simulink model "sim_quadrotor"  (R2015a)
settings: Solver=ode3  StartTime=0  StopTime=40  FixedStep=sampleTime_qcsim  MaxStep=0.1  RelTol=1e-3
InitFcn:
  | % load parameters of the default quadrotor
  | disp('Quadrotor parameters loaded by InitFcn')
  | paramsFilters %load mdl_quadcopter as well!
  | 
  | % change to Simulation folder if in data folder
  | cd([matlabpath '/Simulation']);
values from neighbouring files (symbols this model uses):
  K_lqr_toMotorcmd = lqr(A,B,Q,R)    [LQRControl.m]
undefined symbols (not defined in the file or in its folder): altEstim, controlParams, Discrete, K_poleplace, ofhandle, quad, quadEDT, sampleTime_qcsim, Time, vishandle
libraries: simulink x29, ctrlSharedLib x3, commnoisgen2 x1
(part 2 of 2)

== system sim_quadrotor/DroneRS_Compensator/ControllerFSFB/SysteminputConverter/Takeoffphase_Thrustadjustment ==
  note: NOTE: Below 40cm in altitude, sonar measurements and camera data are very unreliable.
      | We therefore introduce a take-off phase where the drone controls attitude only and runs an uncontrolled total thrust of takeofff_Gain/100  % above equilibrium thrust.
  takeoffphase_flagin : Inport
  totThrustbyController_refin : Inport  Port=2
  Add1 : Sum  Inputs=++|
  HoverThrustLinearizationPoint : Constant  Value=-quad.g*quad.M
  "SCOPE_totalthrust " : Scope
  SaturationThrust : Saturate  UpperLimit=controlParams.totalThrust_maxRelative*controlParams.motorsThrust_i_UpperLimit*4  LowerLimit=-(controlParams.totalThrust_maxRelative*controlParams.motorsThrust_i_UpperLimit*4)
  TakeoffOrControl_Switch : Switch  Criteria=u2 > Threshold
  takeoff_Gain : Gain  Gain=controlParams.takeoff_Gain
  totThrust_refout : Outport
  wires:
  takeoffphase_flagin/1 -> TakeoffOrControl_Switch/2
  SaturationThrust/1 -> totThrust_refout/1, "SCOPE_totalthrust "/1
  TakeoffOrControl_Switch/1 -> Add1/2
  takeoff_Gain/1 -> TakeoffOrControl_Switch/1
  HoverThrustLinearizationPoint/1 -> Add1/1, takeoff_Gain/1
  totThrustbyController_refin/1 -> TakeoffOrControl_Switch/3
  Add1/1 -> SaturationThrust/1

== system sim_quadrotor/DroneRS_Compensator/ControllerFSFB/SysteminputConverter/Thrust2Motorcmd ==
  note: NOTE: This block translates thrust per motor into a command that is acutally send to the motors.
  thrust_refin : Inport
  MotorsRotationDirection : Gain  Gain=[-1,1,-1,1]
  Signed Sqrt : Sqrt  Operator=signedSqrt  SaturateOnIntegerOverflow=on
  ThrustToW2_Gain : Gain  Gain=1/(quad.Ct*quad.rho*quad.A*quad.r^2)
  W2ToMotorsCmd_Gain : Gain  Gain=1/quadEDT.motorsRSToW2_Gain
  motors_cmdout : Outport
  wires:
  MotorsRotationDirection/1 -> W2ToMotorsCmd_Gain/1, Signed Sqrt/1
  Signed Sqrt/1 -> ?  "w"
  W2ToMotorsCmd_Gain/1 -> motors_cmdout/1
  thrust_refin/1 -> ThrustToW2_Gain/1
  ThrustToW2_Gain/1 -> MotorsRotationDirection/1

== system sim_quadrotor/DroneRS_Compensator/ControllerLQR/SysteminputConverter/ControlMixerRS ==
  note: NOTE: The controlmixer translates total thrust and the three torque inputs that the controller came up with into 'thrust per motor'.
  T_refin : Inport
  Qyaw_refin : Inport  Port=2
  Qpitch_refin : Inport  Port=3
  Qroll_refin : Inport  Port=4
  Mux2 : Mux
  Product : Product  Multiplication=Matrix(*)  RndMeth=Zero
  Saturation2 : Saturate  UpperLimit=-0.0118  LowerLimit=-0.3235
  TorquetotalThrustToThrustperMotor : Constant  Value=controlParams.Q2Ts
  thrust_refout : Outport
  wires:
  Qroll_refin/1 -> Mux2/4
  Qpitch_refin/1 -> Mux2/3
  Qyaw_refin/1 -> Mux2/2
  T_refin/1 -> Mux2/1
  Product/1 -> Saturation2/1
  TorquetotalThrustToThrustperMotor/1 -> Product/1
  Mux2/1 -> Product/2
  Saturation2/1 -> thrust_refout/1

== system sim_quadrotor/DroneRS_Compensator/ControllerLQR/SysteminputConverter/Conversion Motorcommands To TotalThrust and Torques ==
  motors_cmdin : Inport
  MotorsRotationDirection : Gain  Gain=diag([-1,1,-1,1])  Multiplication=Matrix(K*u)
  ThrustperMotor To TotalThrust and Torques : Gain  Gain=controlParams.Ts2Q  Multiplication=Matrix(K*u)
  W2ToThrust : Gain  Gain=quad.Ct*quad.rho*quad.A*quad.r^2
  motorsRSToW2_Gain : Gain  Gain=quadEDT.motorsRSToW2_Gain
  u_tthrust_torques : Outport
  wires:
  ThrustperMotor To TotalThrust and Torques/1 -> u_tthrust_torques/1
  motors_cmdin/1 -> MotorsRotationDirection/1
  W2ToThrust/1 -> ThrustperMotor To TotalThrust and Torques/1
  motorsRSToW2_Gain/1 -> W2ToThrust/1
  MotorsRotationDirection/1 -> motorsRSToW2_Gain/1

== system sim_quadrotor/DroneRS_Compensator/ControllerLQR/SysteminputConverter/Takeoffphase_Thrustadjustment ==
  note: NOTE: Below 40cm in altitude, sonar measurements and camera data are very unreliable.
      | We therefore introduce a take-off phase where the drone controls attitude only and runs an uncontrolled total thrust of takeofff_Gain/100  % above equilibrium thrust.
  takeoffphase_flagin : Inport
  totThrustbyController_refin : Inport  Port=2
  Add1 : Sum  Inputs=++|
  HoverThrustLinearizationPoint : Constant  Value=-quad.g*quad.M
  "SCOPE_totalthrust " : Scope
  SaturationThrust : Saturate  UpperLimit=controlParams.totalThrust_maxRelative*controlParams.motorsThrust_i_UpperLimit*4  LowerLimit=-(controlParams.totalThrust_maxRelative*controlParams.motorsThrust_i_UpperLimit*4)
  TakeoffOrControl_Switch : Switch  Criteria=u2 > Threshold
  takeoff_Gain : Gain  Gain=controlParams.takeoff_Gain
  totThrust_refout : Outport
  wires:
  takeoffphase_flagin/1 -> TakeoffOrControl_Switch/2
  SaturationThrust/1 -> totThrust_refout/1, "SCOPE_totalthrust "/1
  TakeoffOrControl_Switch/1 -> Add1/2
  takeoff_Gain/1 -> TakeoffOrControl_Switch/1
  HoverThrustLinearizationPoint/1 -> Add1/1, takeoff_Gain/1
  totThrustbyController_refin/1 -> TakeoffOrControl_Switch/3
  Add1/1 -> SaturationThrust/1

== system sim_quadrotor/DroneRS_Compensator/ControllerLQR/SysteminputConverter/Thrust2Motorcmd ==
  note: NOTE: This block translates thrust per motor into a command that is acutally send to the motors.
  thrust_refin : Inport
  MotorsRotationDirection : Gain  Gain=[-1,1,-1,1]
  Signed Sqrt : Sqrt  Operator=signedSqrt  SaturateOnIntegerOverflow=on
  ThrustToW2_Gain : Gain  Gain=1/(quad.Ct*quad.rho*quad.A*quad.r^2)
  W2ToMotorsCmd_Gain : Gain  Gain=1/quadEDT.motorsRSToW2_Gain
  motors_cmdout : Outport
  wires:
  MotorsRotationDirection/1 -> W2ToMotorsCmd_Gain/1, Signed Sqrt/1
  Signed Sqrt/1 -> ?  "w"
  W2ToMotorsCmd_Gain/1 -> motors_cmdout/1
  thrust_refin/1 -> ThrustToW2_Gain/1
  ThrustToW2_Gain/1 -> MotorsRotationDirection/1

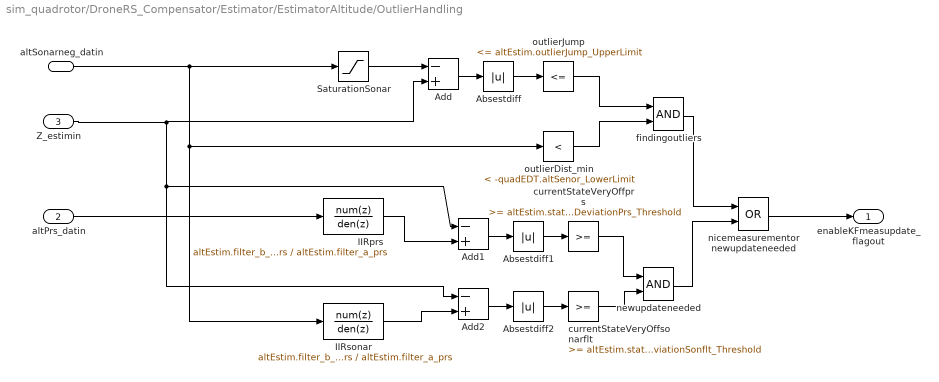
== system sim_quadrotor/DroneRS_Compensator/Estimator/EstimatorAltitude/OutlierHandling ==
  altSonarneg_datin : Inport
  altPrs_datin : Inport  Port=2
  Z_estimin : Inport  Port=3
  Absestdiff : Abs
  Absestdiff1 : Abs
  Absestdiff2 : Abs
  Add : Sum  Inputs=-+
  Add1 : Sum  Inputs=-+
  Add2 : Sum  Inputs=-+
  IIRprs : DiscreteFilter  Numerator=altEstim.filter_b_prs  Denominator=altEstim.filter_a_prs
  IIRsonar : DiscreteFilter  Numerator=altEstim.filter_b_prs  Denominator=altEstim.filter_a_prs
  SaturationSonar : Saturate  UpperLimit=-quadEDT.altSenor_LowerLimit  LowerLimit=-inf
  currentStateVeryOffprs : simulink/Logic and Bit Operations/Compare To Constant  relop=>=  const=altEstim.stateDeviationPrs_Threshold  OutDataTypeStr=boolean
  currentStateVeryOffsonarflt : simulink/Logic and Bit Operations/Compare To Constant  relop=>=  const=altEstim.stateDeviationSonflt_Threshold  OutDataTypeStr=boolean
  findingoutliers : Logic  AllPortsSameDT=off  OutDataTypeStr=boolean
  newupdateneeded : Logic  AllPortsSameDT=off  OutDataTypeStr=boolean
  nicemeasurementor newupdateneeded : Logic  Operator=OR  AllPortsSameDT=off  OutDataTypeStr=boolean
  outlierDist_min : simulink/Logic and Bit Operations/Compare To Constant  relop=<  const=-quadEDT.altSenor_LowerLimit  OutDataTypeStr=boolean
  outlierJump : simulink/Logic and Bit Operations/Compare To Constant  relop=<=  const=altEstim.outlierJump_UpperLimit  OutDataTypeStr=boolean
  enableKFmeasupdate_flagout : Outport
  wires:
  Absestdiff1/1 -> currentStateVeryOffprs/1
  IIRsonar/1 -> Add2/2
  altPrs_datin/1 -> IIRprs/1
  IIRprs/1 -> Add1/2
  currentStateVeryOffsonarflt/1 -> newupdateneeded/2
  Add2/1 -> Absestdiff2/1
  Z_estimin/1 -> Add2/1, Add1/1, Add/2
  currentStateVeryOffprs/1 -> newupdateneeded/1
  altSonarneg_datin/1 -> outlierDist_min/1, IIRsonar/1, SaturationSonar/1
  Absestdiff2/1 -> currentStateVeryOffsonarflt/1
  newupdateneeded/1 -> nicemeasurementor newupdateneeded/2
  Add/1 -> Absestdiff/1
  Absestdiff/1 -> outlierJump/1
  SaturationSonar/1 -> Add/1
  outlierJump/1 -> findingoutliers/1
  outlierDist_min/1 -> findingoutliers/2
  findingoutliers/1 -> nicemeasurementor newupdateneeded/1
  nicemeasurementor newupdateneeded/1 -> enableKFmeasupdate_flagout/1
  Add1/1 -> Absestdiff1/1

== system sim_quadrotor/DroneRS_Compensator/Estimator/EstimatorXYPosition/EstimatorVelocity ==
  opticalFlow_datin : Inport
  Z_estimin : Inport  Port=2
  sensorIMU_datin : Inport  Port=3
  att_estimin : Inport  Port=4
  AccelerationWorld : Subsystem
  Delay : Delay  DelayLength=1  InitialCondition=0
  KalmanFilter_dxdy : ctrlSharedLib/Kalman Filter  TimeDomain=Discrete-Time  UseCurrentEstimator=on  ModelSource=Individual A, B, C, D matrices  ModelSourceVariable=ss(0.95,1,1,0,1)  A=eye(2)  B=sampleTime_qcsim*eye(2)  C=eye(2)  D=0  NumberOfStates=1  NumberOfInputs=1  NumberOfOutputs=1  InitialEstimateSource=Dialog  X0=0  P0=10  UseK=off  UseGH=on  NumberOfProcessNoiseInputs=1  G=eye(2)  TimeInvariantG=on  H=0  TimeInvariantH=on  Q=0.09.*eye(2)  TimeInvariantQ=on  R=5*eye(2)  TimeInvariantR=on  N=0  TimeInvariantN=on  AddInputPort=on  AddEnablePort=on  OutputEstimatedY=off  OutputP=off  Ts=-1
  Mux : Mux  Inputs=2
  OutlierHandling : Subsystem
  SCOPEdxy : Scope
      settings: TimeRange=2.5  YMin=-12  YMax=6
  SCOPEenableKFdxupdate : Scope
      settings: TimeRange=2.2  YMin=0  YMax=1
  SelectplanarOF : Selector  InputPortWidth=3  Indices=[1 2]
  opticalFlowToVelocity_Gain : Gain  Gain=1/quadEDT.VelocityToOpticalFlow_Gain
  dxy_estimout : Outport
  wires:
  att_estimin/1 -> OutlierHandling/1(att_estimin), AccelerationWorld/1(att_estimin)
  sensorIMU_datin/1 -> AccelerationWorld/2(sensorIMU_datin), OutlierHandling/2(sensorIMU_datin)
  opticalFlow_datin/1 -> opticalFlowToVelocity_Gain/1
  SelectplanarOF/1 -> OutlierHandling/4(dxy_estimin), KalmanFilter_dxdy/2, Mux/1
  opticalFlowToVelocity_Gain/1 -> SelectplanarOF/1
  KalmanFilter_dxdy/1 -> Mux/2, dxy_estimout/1, Delay/1
  OutlierHandling/1(Enable_flag) -> SCOPEenableKFdxupdate/1, KalmanFilter_dxdy/3
  Z_estimin/1 -> OutlierHandling/3(Z_estimin)
  Mux/1 -> SCOPEdxy/1
  AccelerationWorld/1(accelerationWorld) -> KalmanFilter_dxdy/1
  Delay/1 -> OutlierHandling/5(dxyOF_datin)

== system sim_quadrotor/DroneRS_Compensator/Estimator/EstimatorXYPosition/EstimatorXYPosition ==
  dxy_estimin : Inport
  att_estimin : Inport  Port=2
  controlModePosVSAtt_flagin : Inport  Port=3
  dz_estimin : Inport  Port=4
  posVIS_datin : Inport  Port=5
  usePosVIS_flagin : Inport  Port=6
  Delay : Delay  DelayLength=1  InitialCondition=0
  KalmanFilter_posxy : ctrlSharedLib/Kalman Filter  TimeDomain=Discrete-Time  UseCurrentEstimator=on  ModelSource=Individual A, B, C, D matrices  ModelSourceVariable=ss(0.95,1,1,0,1)  A=eye(2)  B=sampleTime_qcsim*eye(2)  C=eye(2)  D=0  NumberOfStates=1  NumberOfInputs=1  NumberOfOutputs=1  InitialEstimateSource=Dialog  X0=[.1 0.0]  P0=10  UseK=off  UseGH=on  NumberOfProcessNoiseInputs=1  G=0.1*eye(2)  TimeInvariantG=on  H=0  TimeInvariantH=on  Q=0.001*eye(2)  TimeInvariantQ=on  R=0.3*eye(2)  TimeInvariantR=on  N=0  TimeInvariantN=on  AddInputPort=on  AddEnablePort=on  OutputEstimatedY=off  OutputP=off  Ts=-1
  Mux2 : Mux  Inputs=2
  OutlierHandling : Subsystem
  RStoWorld : MATLAB Function  TreatAsAtomicUnit=on
  SelectXY : Selector  InputPortWidth=4  Indices=[1 2]
  SelectdXY : Selector  InputPortWidth=3  Indices=[1 2]
  SimplyIntegrateVelocity : DiscreteIntegrator  ExternalReset=rising  InitialConditionSetting=State (most efficient)  SampleTime=sampleTime_qcsim  LimitOutput=on  UpperSaturationLimit=2  LowerSaturationLimit=-2
  UseIPPosSwitch : Switch  Criteria=u2 > Threshold
  XY_estimout : Outport
  wires:
  att_estimin/1 -> RStoWorld/1(attitude), OutlierHandling/1(att_estimin)
  dxy_estimin/1 -> Mux2/1
  SimplyIntegrateVelocity/1 -> UseIPPosSwitch/3
  dz_estimin/1 -> Mux2/2
  Mux2/1 -> RStoWorld/2(vector)
  RStoWorld/1(vel_world) -> SelectdXY/1
  SelectdXY/1 -> KalmanFilter_posxy/1, SimplyIntegrateVelocity/1
  posVIS_datin/1 -> SelectXY/1, OutlierHandling/2(posVIS_datin)
  KalmanFilter_posxy/1 -> Delay/1, UseIPPosSwitch/1
  controlModePosVSAtt_flagin/1 -> SimplyIntegrateVelocity/2
  UseIPPosSwitch/1 -> XY_estimout/1
  usePosVIS_flagin/1 -> UseIPPosSwitch/2
  SelectXY/1 -> KalmanFilter_posxy/2
  OutlierHandling/1(enable_flag) -> KalmanFilter_posxy/3
  Delay/1 -> OutlierHandling/3(pos_estim)

== system sim_quadrotor/DroneRS_Compensator/Estimator/EstimatorXYPosition/EstimatorVelocity/AccelerationWorld ==
  note: selectaccelero
  att_estimin : Inport
  sensorIMU_datin : Inport  Port=2
  Add : Sum  Inputs=-+
  Bus Selector1 : BusSelector  OutputSignals=ddx,ddy,ddz
  Mux6 : Mux  Inputs=3
  SelectPlanarddxy : Selector  InputPortWidth=3  Indices=[1 2]
  World2Body : MATLAB Function  TreatAsAtomicUnit=on
  gainaccinput : Gain  Gain=0.2
  gravity : Constant  Value=[0 0 -quad.g]
  accelerationWorld : Outport
  wires:
  att_estimin/1 -> World2Body/1(attitude)
  Bus Selector1/2 -> Mux6/2  "<ddy>"
  Mux6/1 -> Add/2
  sensorIMU_datin/1 -> Bus Selector1/1
  Bus Selector1/1 -> Mux6/1  "<ddx>"
  Bus Selector1/3 -> Mux6/3  "<ddz>"
  SelectPlanarddxy/1 -> gainaccinput/1
  gainaccinput/1 -> accelerationWorld/1
  gravity/1 -> World2Body/2(vector)
  World2Body/1(y) -> Add/1
  Add/1 -> SelectPlanarddxy/1

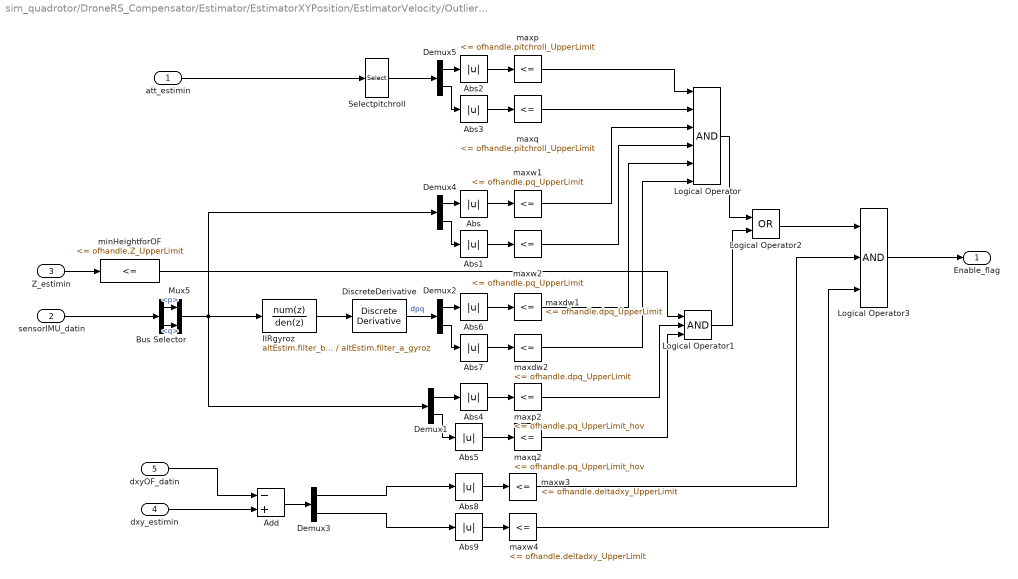
== system sim_quadrotor/DroneRS_Compensator/Estimator/EstimatorXYPosition/EstimatorVelocity/OutlierHandling ==
  att_estimin : Inport
  sensorIMU_datin : Inport  Port=2
  Z_estimin : Inport  Port=3
  dxy_estimin : Inport  Port=4
  dxyOF_datin : Inport  Port=5
  Abs{,1..9} (10 alike) : Abs
  Add : Sum  Inputs=-+
  Bus Selector : BusSelector  OutputSignals=p,q
  Demux{1..5} (5 alike) : Demux  Outputs=2
  DiscreteDerivative : simulink/Discrete/Discrete Derivative  gainval=1.0  ICPrevScaledInput=0.0  InputProcessing=Inherited  OutMin=[]  OutMax=[]  OutDataType=fixdt(1, 16)  OutScaling=2^-10  DoSatur=off
  IIRgyroz : DiscreteFilter  Numerator=altEstim.filter_b_gyroz  Denominator=altEstim.filter_a_gyroz
  Logical Operator : Logic  Inputs=6  AllPortsSameDT=off  OutDataTypeStr=boolean
  Logical Operator1 : Logic  Inputs=3  AllPortsSameDT=off  OutDataTypeStr=boolean
  Logical Operator2 : Logic  Operator=OR  AllPortsSameDT=off  OutDataTypeStr=boolean
  Logical Operator3 : Logic  Inputs=3  AllPortsSameDT=off  OutDataTypeStr=boolean
  Mux5 : Mux  Inputs=2
  Selectpitchroll : Selector  InputPortWidth=3  Indices=[2 3]
  maxdw1 : simulink/Logic and Bit Operations/Compare To Constant  relop=<=  const=ofhandle.dpq_UpperLimit  OutDataTypeStr=boolean
  maxdw2 : simulink/Logic and Bit Operations/Compare To Constant  relop=<=  const=ofhandle.dpq_UpperLimit  OutDataTypeStr=boolean
  maxp : simulink/Logic and Bit Operations/Compare To Constant  relop=<=  const=ofhandle.pitchroll_UpperLimit  OutDataTypeStr=boolean
  maxp2 : simulink/Logic and Bit Operations/Compare To Constant  relop=<=  const=ofhandle.pq_UpperLimit_hov  OutDataTypeStr=boolean
  maxq : simulink/Logic and Bit Operations/Compare To Constant  relop=<=  const=ofhandle.pitchroll_UpperLimit  OutDataTypeStr=boolean
  maxq2 : simulink/Logic and Bit Operations/Compare To Constant  relop=<=  const=ofhandle.pq_UpperLimit_hov  OutDataTypeStr=boolean
  maxw1 : simulink/Logic and Bit Operations/Compare To Constant  relop=<=  const=ofhandle.pq_UpperLimit  OutDataTypeStr=boolean
  maxw2 : simulink/Logic and Bit Operations/Compare To Constant  relop=<=  const=ofhandle.pq_UpperLimit  OutDataTypeStr=boolean
  maxw3 : simulink/Logic and Bit Operations/Compare To Constant  relop=<=  const=ofhandle.deltadxy_UpperLimit  OutDataTypeStr=boolean
  maxw4 : simulink/Logic and Bit Operations/Compare To Constant  relop=<=  const=ofhandle.deltadxy_UpperLimit  OutDataTypeStr=boolean
  minHeightforOF : simulink/Logic and Bit Operations/Compare To Constant  relop=<=  const=ofhandle.Z_UpperLimit  OutDataTypeStr=boolean
  Enable_flag : Outport
  wires:
  maxp2/1 -> Logical Operator1/2
  Demux5/2 -> Abs3/1
  minHeightforOF/1 -> Logical Operator1/1
  Demux5/1 -> Abs2/1
  maxq/1 -> Logical Operator/2
  maxdw2/1 -> Logical Operator/6
  maxdw1/1 -> Logical Operator/5
  att_estimin/1 -> Selectpitchroll/1
  maxw2/1 -> Logical Operator/4
  maxp/1 -> Logical Operator/1
  Bus Selector/2 -> Mux5/2  "<q>"
  maxq2/1 -> Logical Operator1/3
  sensorIMU_datin/1 -> Bus Selector/1
  Selectpitchroll/1 -> Demux5/1
  Bus Selector/1 -> Mux5/1  "<p>"
  maxw1/1 -> Logical Operator/3
  Logical Operator/1 -> Logical Operator2/1
  Z_estimin/1 -> minHeightforOF/1
  Abs/1 -> maxw1/1
  Abs1/1 -> maxw2/1
  Demux4/1 -> Abs/1
  Demux4/2 -> Abs1/1
  Abs2/1 -> maxp/1
  Abs3/1 -> maxq/1
  Abs4/1 -> maxp2/1
  Abs5/1 -> maxq2/1
  Demux1/1 -> Abs4/1
  Demux1/2 -> Abs5/1
  Logical Operator1/1 -> Logical Operator2/2
  Abs6/1 -> maxdw1/1
  Abs7/1 -> maxdw2/1
  Demux2/1 -> Abs6/1
  Demux2/2 -> Abs7/1
  DiscreteDerivative/1 -> Demux2/1  "dpq"
  Logical Operator3/1 -> Enable_flag/1
  Logical Operator2/1 -> Logical Operator3/1
  Abs8/1 -> maxw3/1
  Abs9/1 -> maxw4/1
  Add/1 -> Demux3/1
  dxy_estimin/1 -> Add/2
  Demux3/1 -> Abs8/1
  Demux3/2 -> Abs9/1
  dxyOF_datin/1 -> Add/1
  maxw3/1 -> Logical Operator3/2
  maxw4/1 -> Logical Operator3/3
  Mux5/1 -> Demux4/1, Demux1/1, IIRgyroz/1
  IIRgyroz/1 -> DiscreteDerivative/1

== system sim_quadrotor/DroneRS_Compensator/Estimator/EstimatorXYPosition/EstimatorXYPosition/OutlierHandling ==
  att_estimin : Inport
  posVIS_datin : Inport  Port=2
  pos_estim : Inport  Port=3
  Add1 : Sum  Inputs=+-
  Demux6 : Demux  Outputs=3
  Logical Operator3 : Logic  Inputs=4  AllPortsSameDT=off  OutDataTypeStr=boolean
  SelectX : Selector  InputPortWidth=4  Indices=[1]
  SelectXY : Selector  InputPortWidth=4  Indices=[1 2]
  abs : MATLAB Function  TreatAsAtomicUnit=on
  checkPosavailable : simulink/Logic and Bit Operations/Compare To Constant  relop=~=  const=-99  OutDataTypeStr=boolean
  maxp3 : simulink/Logic and Bit Operations/Compare To Constant  relop=<=  const=vishandle.att_UpperLimit  OutDataTypeStr=boolean
  maxq3 : simulink/Logic and Bit Operations/Compare To Constant  relop=<=  const=vishandle.att_UpperLimit  OutDataTypeStr=boolean
  planarjumpsVISPOS : simulink/Logic and Bit Operations/Compare To Constant  relop=<  const=vishandle.deltaXY  OutDataTypeStr=boolean
  enable_flag : Outport
  wires:
  att_estimin/1 -> Demux6/1
  posVIS_datin/1 -> SelectXY/1, SelectX/1
  SelectX/1 -> checkPosavailable/1
  checkPosavailable/1 -> Logical Operator3/1
  Logical Operator3/1 -> enable_flag/1
  Demux6/2 -> maxp3/1
  Demux6/3 -> maxq3/1
  maxp3/1 -> Logical Operator3/2
  maxq3/1 -> Logical Operator3/3
  SelectXY/1 -> Add1/1
  Add1/1 -> abs/1(vec)
  pos_estim/1 -> Add1/2
  abs/1(y) -> planarjumpsVISPOS/1
  planarjumpsVISPOS/1 -> Logical Operator3/4

== matlab function sim_quadrotor/Drone_Sensorsystem/camera/trafo_RTB2RSSensors_trans ==
  data: u input; y output
function y = fcn(u)
%inverse yaw-rotation
y = ([cos(pi/4) sin(pi/4) 0 ; -sin(pi/4) cos(pi/4) 0; 0 0 1]*u);

== matlab function sim_quadrotor/DroneRS_Compensator/ControllerPID2W/inverse rotation Function ==
  data: u input; y output
function y = fcn(u)
%inverse yaw-rotation
y = ([cos(u) sin(u); -sin(u) cos(u)]);

== matlab function sim_quadrotor/Drone_Sensorsystem/IMU_Pressure/trafo_RTB2RSSensors_trans ==
  data: u input; y output
function y = fcn(u)
%inverse yaw-rotation
y = ([cos(pi/4) sin(pi/4) 0 ; -sin(pi/4) cos(pi/4) 0; 0 0 1]*u);

== matlab function sim_quadrotor/Drone_Sensorsystem/IMU_Pressure/trafo_RTB2World_trans ==
  data: attitude input; vector input; y output
function y = fcn(attitude,vector)

yaw = attitude(1);
pitch = attitude(2);
roll = attitude(3);

R_RTBBody2Global =[ [ cos(pitch)*cos(yaw), cos(yaw)*sin(pitch)*sin(roll) - cos(roll)*sin(yaw), sin(roll)*sin(yaw) + cos(roll)*cos(yaw)*sin(pitch)];
[ cos(pitch)*sin(yaw), cos(roll)*cos(yaw) + sin(pitch)*sin(roll)*sin(yaw), cos(roll)*sin(pitch)*sin(yaw) - cos(yaw)*sin(roll)];
[         -sin(pitch),                               cos(pitch)*sin(roll),                               cos(pitch)*cos(roll)]];

% Rw_Global2RTBBody  = [0        sin(roll)          cos(roll);             %inverted Wronskian
%           0        cos(roll)*cos(pitch) -sin(roll)*cos(pitch);
%           cos(pitch) sin(roll)*sin(pitch) cos(roll)*sin(pitch)] / cos(pitch);
      
      
      
 y = R_RTBBody2Global*vector;      
      
%y = -([cos(pi/4) sin(pi/4); -sin(pi/4) cos(pi/4)]*u);

== matlab function sim_quadrotor/Drone_Sensorsystem/IMU_Pressure/trafo_World2RTB_trans1 ==
  data: attitude input; vector input; y output
function y = fcn(attitude,vector)

yaw = attitude(1);
pitch = attitude(2);
roll = attitude(3);

R_Global2RTBBody = [[                                cos(pitch)*cos(yaw),                                cos(pitch)*sin(yaw),          -sin(pitch)];
                    [ cos(yaw)*sin(pitch)*sin(roll) - cos(roll)*sin(yaw), cos(roll)*cos(yaw) + sin(pitch)*sin(roll)*sin(yaw), cos(pitch)*sin(roll)];
                    [ sin(roll)*sin(yaw) + cos(roll)*cos(yaw)*sin(pitch), cos(roll)*sin(pitch)*sin(yaw) - cos(yaw)*sin(roll), cos(pitch)*cos(roll)]];


% Rw_Global2RTBBody  = [0        sin(roll)          cos(roll);             %inverted Wronskian
%           0        cos(roll)*cos(pitch) -sin(roll)*cos(pitch);
%           cos(pitch) sin(roll)*sin(pitch) cos(roll)*sin(pitch)] / cos(pitch);
      
      
      
 y = R_Global2RTBBody*vector;      
      
%y = -([cos(pi/4) sin(pi/4); -sin(pi/4) cos(pi/4)]*u);

== matlab function sim_quadrotor/Drone_Sensorsystem/IMU_Pressure/trafo_RTB2RSSensors_rot1 ==
  data: u input; y output
function y = fcn(u)
%inverse yaw-rotation
y = [cos(pi/4)  sin(pi/4); -sin(pi/4) cos(pi/4)]*u;

== matlab function sim_quadrotor/DroneRS_Compensator/Estimator/EstimatorXYPosition/EstimatorVelocity/AccelerationWorld/World2Body ==
  data: attitude input; vector input; y output
function y = fcn(attitude,vector)

yaw = attitude(1);
pitch = attitude(2);
roll = attitude(3);

% rotz(yaw)*roty(pitch)*rotx(roll)
%     R_RTBBodytoGlobal = [cos(pitch)*cos(yaw) sin(roll)*sin(pitch)*cos(yaw)-cos(roll)*sin(yaw) cos(roll)*sin(pitch)*cos(yaw)+sin(roll)*sin(yaw);   %BBF > Inertial rotation matrix
%          cos(pitch)*sin(yaw) sin(roll)*sin(pitch)*sin(yaw)+cos(roll)*cos(yaw) cos(roll)*sin(pitch)*sin(yaw)-sin(roll)*cos(yaw);
%          -sin(pitch)         sin(roll)*cos(pitch)                            cos(roll)*cos(pitch)];
    

R_Global2RTBBody = [[                                cos(pitch)*cos(yaw),                                cos(pitch)*sin(yaw),          -sin(pitch)];
                    [ cos(yaw)*sin(pitch)*sin(roll) - cos(roll)*sin(yaw), cos(roll)*cos(yaw) + sin(pitch)*sin(roll)*sin(yaw), cos(pitch)*sin(roll)];
                    [ sin(roll)*sin(yaw) + cos(roll)*cos(yaw)*sin(pitch), cos(roll)*sin(pitch)*sin(yaw) - cos(yaw)*sin(roll), cos(pitch)*cos(roll)]];

% Rw_Global2RTBBody  = [0        sin(roll)          cos(roll);             %inverted Wronskian
%           0        cos(roll)*cos(pitch) -sin(roll)*cos(pitch);
%           cos(pitch) sin(roll)*sin(pitch) cos(roll)*sin(pitch)] / cos(pitch);
      
      
      
 y = R_Global2RTBBody*vector;      
      
%y = -([cos(pi/4) sin(pi/4); -sin(pi/4) cos(pi/4)]*u);

== matlab function sim_quadrotor/DroneRS_Compensator/Estimator/EstimatorXYPosition/EstimatorXYPosition/RStoWorld ==
  data: attitude input; vector input; vel_world output
function vel_world = fcn(attitude,vector)
yaw = attitude(1);
pitch = attitude(2);
roll = attitude(3);








R_RTBBodytoGlobal = [cos(pitch)*cos(yaw) sin(roll)*sin(pitch)*cos(yaw)-cos(roll)*sin(yaw) cos(roll)*sin(pitch)*cos(yaw)+sin(roll)*sin(yaw);   %BBF > Inertial rotation matrix
  cos(pitch)*sin(yaw) sin(roll)*sin(pitch)*sin(yaw)+cos(roll)*cos(yaw) cos(roll)*sin(pitch)*sin(yaw)-sin(roll)*cos(yaw);
  -sin(pitch)         sin(roll)*cos(pitch)                            cos(roll)*cos(pitch)];

vel_world = R_RTBBodytoGlobal*vector;

== matlab function sim_quadrotor/DroneRS_Compensator/Estimator/EstimatorAltitude/RStoWorldinacc ==
  data: attitude input; vector input; acc_world output
function acc_world = fcn(attitude,vector)
yaw = attitude(1);
pitch = attitude(2);
roll = attitude(3);








R_RTBBodytoGlobal = [cos(pitch)*cos(yaw) sin(roll)*sin(pitch)*cos(yaw)-cos(roll)*sin(yaw) cos(roll)*sin(pitch)*cos(yaw)+sin(roll)*sin(yaw);   %BBF > Inertial rotation matrix
  cos(pitch)*sin(yaw) sin(roll)*sin(pitch)*sin(yaw)+cos(roll)*cos(yaw) cos(roll)*sin(pitch)*sin(yaw)-sin(roll)*cos(yaw);
  -sin(pitch)         sin(roll)*cos(pitch)                            cos(roll)*cos(pitch)];

acc_world = R_RTBBodytoGlobal*vector;

== matlab function sim_quadrotor/DroneRS_Compensator/Estimator/EstimatorAltitude/WorldToRSinacc ==
  data: attitude input; vector input; acc_RS output
function acc_RS = fcn(attitude,vector)
yaw = attitude(1);
pitch = attitude(2);
roll = attitude(3);


R_Global2RTBBody = [[                                cos(pitch)*cos(yaw),                                cos(pitch)*sin(yaw),          -sin(pitch)];
                    [ cos(yaw)*sin(pitch)*sin(roll) - cos(roll)*sin(yaw), cos(roll)*cos(yaw) + sin(pitch)*sin(roll)*sin(yaw), cos(pitch)*sin(roll)];
                    [ sin(roll)*sin(yaw) + cos(roll)*cos(yaw)*sin(pitch), cos(roll)*sin(pitch)*sin(yaw) - cos(yaw)*sin(roll), cos(pitch)*cos(roll)]];

acc_RS = R_Global2RTBBody*vector;

== matlab function sim_quadrotor/DroneRS_Compensator/Estimator/EstimatorAttitude ==
  data: sensorIMU_datin input; yawVIS_datin input; validVIS_flagin input; gvecInit_datin input; att_estimout output; dt input; datt_estimout output; w_euler output
function [att_estimout,datt_estimout,w_euler] = fcn(sensorIMU_datin,yawVIS_datin,validVIS_flagin, gvecInit_datin,dt)
persistent yaw_cur pitch_cur roll_cur

p = sensorIMU_datin(4);
q = sensorIMU_datin(5);
r = sensorIMU_datin(6);

g = norm(gvecInit_datin,2);

if isempty(yaw_cur)
   yaw_cur = 0;
end
if isempty(pitch_cur)
   pitch_cur = 0;
end
if isempty(roll_cur)
   roll_cur = 0;
end


accvsGyro     = 0.001;
[yaw,pitch,roll,w_euler,forceMagnitudeApprox]= complimentaryfilter(yaw_cur, pitch_cur, roll_cur, g,dt,sensorIMU_datin, yawVIS_datin,validVIS_flagin,accvsGyro);
yaw_cur = yaw;
pitch_cur = pitch;
roll_cur = roll;

att_estimout = [yaw,pitch,roll]';
datt_estimout = [p,q,r]';

== matlab function sim_quadrotor/DroneRS_Compensator/Estimator/EstimatorXYPosition/EstimatorXYPosition/OutlierHandling/abs ==
  data: vec input; y output
function y = fcn(vec)
y = norm(vec,2);
